simulink model "s1"  (R2021b)
settings: Solver=ode45  StartTime=0.0  StopTime=15.0  MaxStep=0.01  RelTol=1e-3
settings Model: Creator=Student  LastModifiedBy=Student

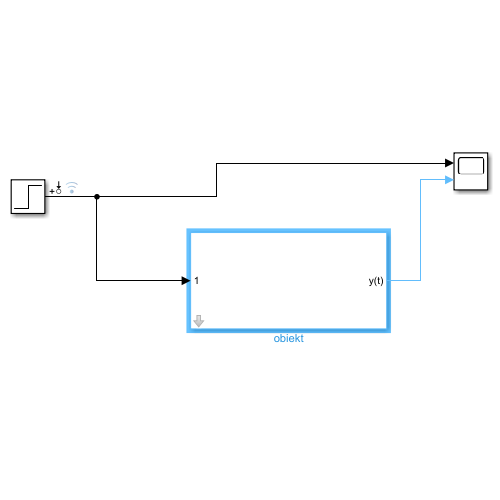
[thumbnail: Simulink's stored preview of the top-level diagram]
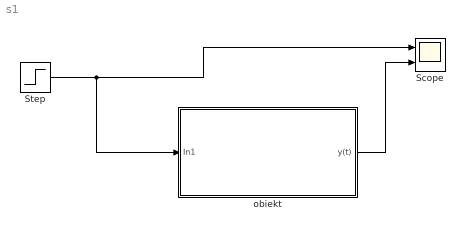
== system s1 ==
  Scope : Scope  NumInputPorts=2
  Step : Step  Time=0  SampleTime=0
  obiekt : Subsystem  mask{wn=1, zeta=0.25}
      mask prompts: wn "wn - czestotliwosc drgan wlasnych"; zeta "zeta - wspolczynnik tlumienia"
  wires:
  Step/1 -> obiekt/1(In1), Scope/1
  obiekt/1(y(t)) -> Scope/2

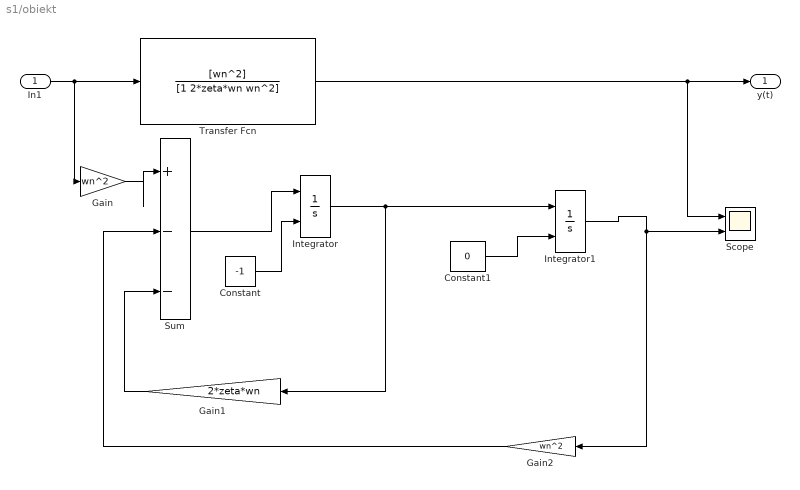
== system s1/obiekt ==
  In1 : Inport
  Constant : Constant  Value=-1
  Constant1 : Constant  Value=0
  Gain : Gain  Gain=wn^2
  Gain1 : Gain  Gain=2*zeta*wn
  Gain2 : Gain  Gain=wn^2
  Integrator : Integrator  InitialConditionSource=external
  Integrator1 : Integrator  InitialConditionSource=external
  Scope : Scope  NumInputPorts=2
  Sum : Sum  Inputs=|+--
  Transfer Fcn : TransferFcn  Numerator=[wn^2]  Denominator=[1 2*zeta*wn wn^2]
  y(t) : Outport
  wires:
  Transfer Fcn/1 -> Scope/1, y(t)/1
  In1/1 -> Gain/1, Transfer Fcn/1
  Gain/1 -> Sum/1
  Constant/1 -> Integrator/2
  Sum/1 -> Integrator/1
  Gain1/1 -> Sum/3
  Integrator/1 -> Gain1/1, Integrator1/1
  Constant1/1 -> Integrator1/2
  Gain2/1 -> Sum/2
  Integrator1/1 -> Scope/2, Gain2/1
